simulink model "TrafficLights"  (R2022a)
settings: Solver=FixedStepAuto  StartTime=0.0  StopTime=inf  FixedStep=0.01  RelTol=1e-3  EnableMultiTasking=on
libraries: arduinolib x3
settings Model: ExtModeTrigDuration=2  Creator=bujji  LastModifiedBy=bujji
settings OptimizationCC: EnhancedBackFolding=on  PassReuseOutputArgsAs=Individual arguments  ZeroExternalMemoryAtStartup=off  ZeroInternalMemoryAtStartup=off  MaxStackSize=64  OptimizeBlockOrder=speed  DifferentSizesBufferReuse=on  OptimizationCustomize=off  EfficientTunableParamExpr=on
settings DebuggingCC: ParameterTunabilityLossMsg=error
settings HardwareCC: ProdBitPerInt=16  ProdBitPerPointer=16  ProdBitPerSizeT=16  ProdBitPerPtrDiffT=16  ProdLargestAtomicFloat=None  ProdWordSize=8  ProdHWDeviceType=Atmel->AVR
settings SFSimCC: MATLABDynamicMemAlloc=off
settings RTWCC: SystemTargetFile=ert.tlc  HardwareBoard=Arduino Mega 2560  TemplateMakefile=ert_default_tmf  Toolchain=Arduino AVR  BuildConfiguration=Faster Runs
settings CodeAppCC: ForceParamTrailComments=on  IgnoreCustomStorageClasses=off  OperatorAnnotations=on  SimulinkDataObjDesc=on  SFDataObjDesc=on  InsertBlockDesc=on
settings ERTTargetCC: SupportContinuousTime=on  SupportVariableSizeSignals=on  ExtModeTransport=3  ExtModeStaticAlloc=on  ExtModeStaticAllocSize=2048  ExtModeMexFile=ext_xcp  ExtModeIntrfLevel=Level2 - Open

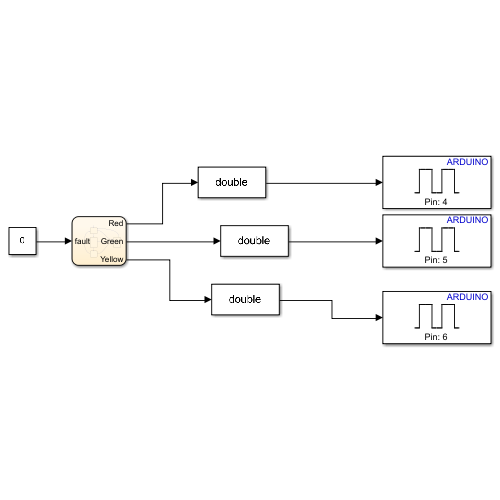
[thumbnail: Simulink's stored preview of the top-level diagram]
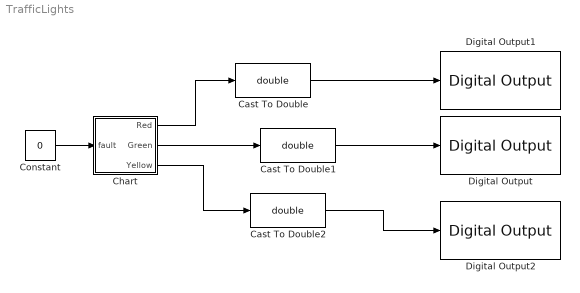
== system TrafficLights ==
  Cast To Double : DataTypeConversion  OutDataTypeStr=double  SaturateOnIntegerOverflow=off  RndMeth=Floor
  Cast To Double1 : DataTypeConversion  OutDataTypeStr=double  SaturateOnIntegerOverflow=off  RndMeth=Floor
  Cast To Double2 : DataTypeConversion  OutDataTypeStr=double  SaturateOnIntegerOverflow=off  RndMeth=Floor
  Chart : Stateflow chart  TreatAsAtomicUnit=on
  Constant : Constant  Value=0
  Digital Output : arduinolib/Digital Output  pinNumber=5  Direction=output  blockPlatform=arduino
  Digital Output1 : arduinolib/Digital Output  pinNumber=4  Direction=output  blockPlatform=arduino
  Digital Output2 : arduinolib/Digital Output  pinNumber=6  Direction=output  blockPlatform=arduino
  wires:
  Chart/2(Green) -> Cast To Double1/1
  Chart/1(Red) -> Cast To Double/1
  Chart/3(Yellow) -> Cast To Double2/1
  Constant/1 -> Chart/1(fault)
  Cast To Double/1 -> Digital Output1/1
  Cast To Double1/1 -> Digital Output/1
  Cast To Double2/1 -> Digital Output2/1

== stateflow chart TrafficLights/Chart ==
  state Red
    entry:
    Red=1;
    Green=0;
    Yellow=0;
  state Green
    entry:
    Red=0;
    Green=1;
    Yellow=0;
  state Fault
    during:
    Red=1;
    Green=0;
    Yellow=0;
  state Yellow
    entry:
    Red=0;
    Green=0;
    Yellow=1;
  (default) -> Red
  Fault -> Red : [fault==0]
  Red -> Fault [order 2] : [fault==1]
  Yellow -> Red [order 1] : after(10,sec)
  Red -> Green [order 1] : after(30,sec)
  Green -> Fault [order 2] : [fault==1]
  Yellow -> Fault [order 2] : [fault==1]
  Green -> Yellow [order 1] : after(60,sec)
  data: fault input; Red output; Green output; Yellow output
